simulink model "Simulacion_Ctrls"  (R2017a)
settings: Solver=VariableStepAuto  StartTime=0.0  StopTime=2  RelTol=1e-3  EnableMultiTasking=on
values from neighbouring files (symbols this model uses):
  Control = K*Num_Comp*Den_Comp*(Polos_1^Num_P1)    [Control_LGR.m]    (also in Control_PID_Discreto.m = F_PID_D)
  den_Planta = [1 56.1 522.8]    [Control_LGR.m]    (also in Control_PID_Discreto.m)
  F_D = c2d(F_C,T,'zoh')    [Control_LGR.m]    (also in Control_PID_Discreto.m)
  num_Planta = [364.4]    [Control_LGR.m]    (also in Control_PID_Discreto.m)
  T = Tsd/10    [Control_LGR.m]    (also in Control_PID_Discreto.m)
settings Model: Creator=-Valentina  LastModifiedBy=ThinaYushiko
settings OptimizationCC: LifeSpan=inf
settings DebuggingCC: SFUnexpectedBacktrackingDiag=warning  SFNoUnconditionalDefaultTransitionDiag=warning  SFExecutionAtInitializationDiag=none
settings GRTTargetCC: TargetLangStandard=C89/C90 (ANSI)  GeneratePreprocessorConditionals=Disable all
settings ConfigComp: CovMetricSettings=dw  CovHtmlReporting=on  CovSaveCumulativeToWorkspaceVar=on  CovSaveSingleToWorkspaceVar=on  CovExternalEMLEnable=off

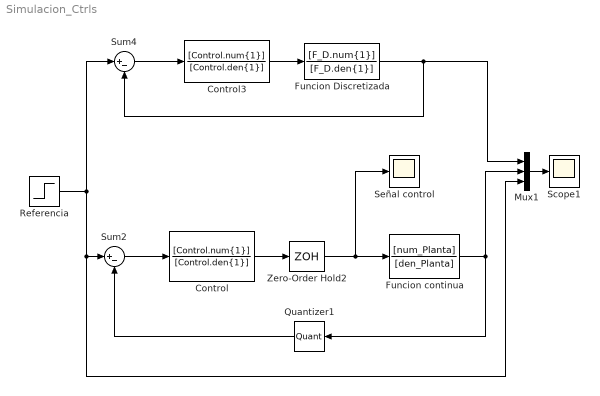
== system Simulacion_Ctrls ==
  Control : DiscreteFilter  Numerator=[Control.num{1}]  Denominator=[Control.den{1}]  SampleTime=T
  Control3 : DiscreteFilter  Numerator=[Control.num{1}]  Denominator=[Control.den{1}]  SampleTime=T
  Funcion Discretizada : DiscreteTransferFcn  Numerator=[F_D.num{1}]  Denominator=[F_D.den{1}]  SampleTime=T
  Funcion continua : TransferFcn  Numerator=[num_Planta]  Denominator=[den_Planta]
  Mux1 : Mux  Inputs=3
  Quantizer1 : Quantizer  QuantizationInterval=1/1024
  Referencia : Step  Time=0  After=200  SampleTime=0
  Scope1 : Scope
  Señal control : Scope
  Sum2 : Sum  Inputs=|+-
  Sum4 : Sum  Inputs=|+-
  Zero-Order Hold2 : ZeroOrderHold  SampleTime=T
  wires:
  Sum2/1 -> Control/1
  Control/1 -> Zero-Order Hold2/1
  Zero-Order Hold2/1 -> Funcion continua/1, Señal control/1
  Quantizer1/1 -> Sum2/2
  Mux1/1 -> Scope1/1
  Funcion continua/1 -> Quantizer1/1, Mux1/2
  Sum4/1 -> Control3/1
  Funcion Discretizada/1 -> Mux1/1, Sum4/2
  Referencia/1 -> Sum4/1, Mux1/3, Sum2/1
  Control3/1 -> Funcion Discretizada/1
